simulink model "DT_Openloop"  (R2015a)
settings: Solver=FixedStepDiscrete  StartTime=0.0  StopTime=Tf  FixedStep=Ts  MaxStep=1e-5  RelTol=1e-4
values from neighbouring files (symbols this model uses):
  A = [0 1; -2 -3]    [sv__feedback__observer_driver.m]    (also in sv__feedback__observer_type1_driver.m; sv__feedback_driver.m; sv__feedback_type1_driver.m; tf_sv_driver.m)
  B = [1; 0]    [sv__feedback__observer_driver.m]    (also in sv__feedback__observer_type1_driver.m; sv__feedback_driver.m; sv__feedback_type1_driver.m; tf_sv_driver.m)
  C = [1 0]    [sv__feedback__observer_driver.m]    (also in sv__feedback__observer_type1_driver.m = [0 1]; sv__feedback_driver.m; sv__feedback_type1_driver.m; tf_sv_driver.m)
  c = 0.968    [wheel_match.m]    (also in wheel_parameters.m = 0.96017)
  Control_effort_saturation = MAX_DUTY*AD_scale/Convert_to_dutycycle    (= 163.68)    [wheel_parameters.m]
  delay = 1    [wheel_match.m]    (also in wheel_parameters.m)
  Falling_slew = -MAX_DELTA_U*AD_scale/(Ts*Convert_to_dutycycle)    (= -111.052310197)    [wheel_parameters.m]
  Max_speed = 113.0    (= 113)    [wheel_parameters.m]
  Relay_off = 14.0    (= 14)    [wheel_parameters.m]
  Relay_on = 26.0    (= 26)    [wheel_parameters.m]
  Rising_slew = MAX_DELTA_U*AD_scale/(Ts*Convert_to_dutycycle)    (= 111.052310197)    [wheel_parameters.m]
  Ts = t(2)-t(1)    [check_filter.m]    (also in closedloop_driver.m = 0.1; openloop_driver.m = 0.1; wheel_parameters.m = 0.05)
settings Model: Creator=throne  LastModifiedBy=throne
settings DataIOCC: SignalLoggingSaveFormat=ModelDataLogs  SignalLoggingName=sigsOut
settings OptimizationCC: ExpressionDepthLimit=2147483647
settings DebuggingCC: SaveWithParameterizedLinksMsg=none  UnderspecifiedInitializationDetection=Classic  MergeDetectMultiDrivingBlocksExec=none  SignalResolutionControl=TryResolveAllWithWarning  MultiTaskDSMMsg=warning  MultiTaskCondExecSysMsg=none  StateNameClashWarn=warning
settings HardwareCC: TargetUnknown=on
settings GRTTargetCC: CombineOutputUpdateFcns=off  GRTInterface=on

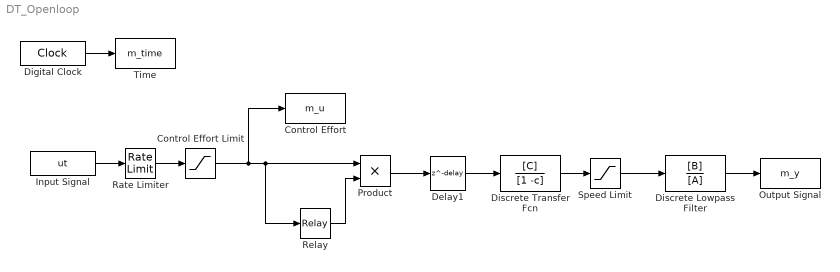
== system DT_Openloop ==
  Control Effort : ToWorkspace  VariableName=m_u  SampleTime=-1
  "Control Effort Limit " : Saturate  UpperLimit=Control_effort_saturation  LowerLimit=0  OutMin=0  OutMax=[Control_effort_saturation]
  Delay1 : Delay  DelayLength=delay  SampleTime=Ts
  Digital Clock : DigitalClock  SampleTime=Ts
  Discrete Lowpass Filter : DiscreteTransferFcn  Numerator=[B]  Denominator=[A]
  Discrete Transfer Fcn : DiscreteTransferFcn  Numerator=[C]  Denominator=[1 -c]  SampleTime=Ts
  "Input Signal " : FromWorkspace  VariableName=ut  SampleTime=Ts
  Output Signal : ToWorkspace  VariableName=m_y  SampleTime=-1
  Product : Product  RndMeth=Zero
  Rate Limiter : RateLimiter  RisingSlewLimit=Rising_slew  FallingSlewLimit=Falling_slew  SampleTimeMode=inherited
  Relay : Relay  OnSwitchValue=Relay_on  OffSwitchValue=Relay_off  SampleTime=Ts
  Speed Limit : Saturate  UpperLimit=Max_speed  LowerLimit=0
  Time : ToWorkspace  VariableName=m_time  SampleTime=-1
  wires:
  Digital Clock/1 -> Time/1
  Relay/1 -> Product/2
  Discrete Transfer Fcn/1 -> Speed Limit/1
  Delay1/1 -> Discrete Transfer Fcn/1
  Speed Limit/1 -> Discrete Lowpass Filter/1
  Discrete Lowpass Filter/1 -> Output Signal/1
  "Input Signal "/1 -> Rate Limiter/1
  Product/1 -> Delay1/1
  Rate Limiter/1 -> "Control Effort Limit "/1
  "Control Effort Limit "/1 -> Control Effort/1, Relay/1, Product/1
